simulink model "Cellmodel"  (Simulink 6.6)
settings: Solver=ode4  StartTime=0.0  StopTime=0.0001  FixedStep=0.000000001  RelTol=1e-3
(part 2 of 2)

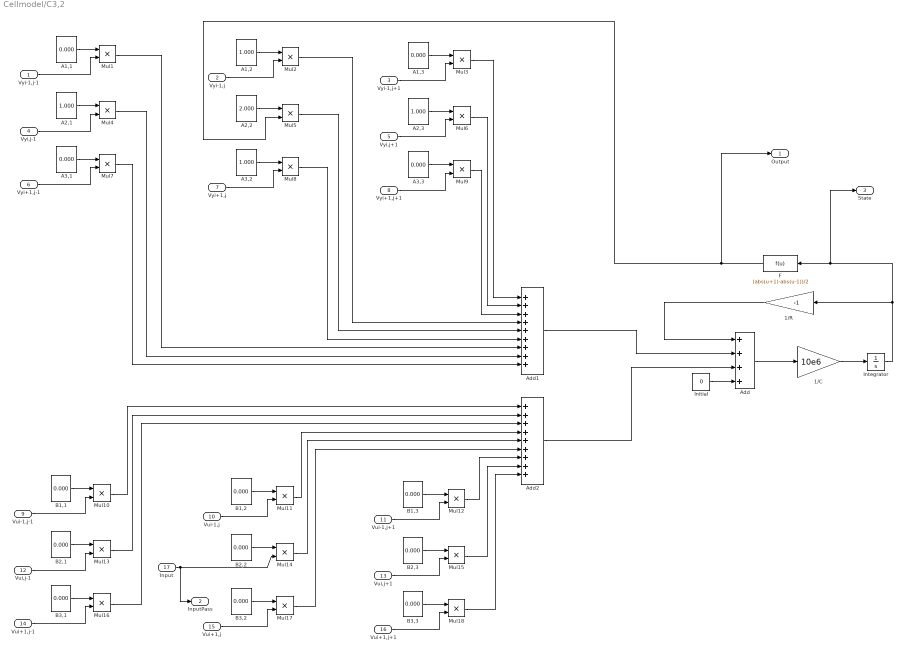
== system Cellmodel/C3,2 ==
  Vyi-1,j-1 : Inport
  Vyi-1,j : Inport  Port=2
  Vyi-1,j+1 : Inport  Port=3
  Vyi,j-1 : Inport  Port=4
  Vyi,j+1 : Inport  Port=5
  Vyi+1,j-1 : Inport  Port=6
  Vyi+1,j : Inport  Port=7
  Vyi+1,j+1 : Inport  Port=8
  Vui-1,j-1 : Inport  Port=9
  Vui-1,j : Inport  Port=10
  Vui-1,j+1 : Inport  Port=11
  Vui,j-1 : Inport  Port=12
  Vui,j+1 : Inport  Port=13
  Vui+1,j-1 : Inport  Port=14
  Vui+1,j : Inport  Port=15
  Vui+1,j+1 : Inport  Port=16
  Input : Inport  Port=17
  1/C : Gain  Gain=10e6
  1/R : Gain  Orientation=left  Gain=-1
  A1,1 : Constant  Value=0.000
  A1,2 : Constant  Value=1.000
  A1,3 : Constant  Value=0.000
  A2,1 : Constant  Value=1.000
  A2,2 : Constant  Value=2.000
  A2,3 : Constant  Value=1.000
  A3,1 : Constant  Value=0.000
  A3,2 : Constant  Value=1.000
  A3,3 : Constant  Value=0.000
  Add : Sum  Inputs=++++  OutScaling=2^-10
  Add1 : Sum  Inputs=+++++++++  OutScaling=2^-10
  Add2 : Sum  Inputs=+++++++++  OutScaling=2^-10
  B1,1 : Constant  Value=0.000
  B1,2 : Constant  Value=0.000
  B1,3 : Constant  Value=0.000
  B2,1 : Constant  Value=0.000
  B2,2 : Constant  Value=0.000
  B2,3 : Constant  Value=0.000
  B3,1 : Constant  Value=0.000
  B3,2 : Constant  Value=0.000
  B3,3 : Constant  Value=0.000
  F : Fcn  Orientation=left  Expr=(abs(u+1)-abs(u-1))/2
  Initial : Constant  Value=0
  Integrator : Integrator  InitialCondition=0.900
  Mul{1..18} (18 alike) : Product  Inputs=**  OutScaling=2^-10
  Output : Outport
  InputPass : Outport  Port=2
  State : Outport  Port=3
  wires:
  Add2/1 -> Add/3
  Input/1 -> InputPass/1, Mul14/2
  Mul18/1 -> Add2/9
  Mul15/1 -> Add2/8
  Mul12/1 -> Add2/7
  Mul17/1 -> Add2/6
  Mul14/1 -> Add2/5
  Mul11/1 -> Add2/4
  Mul16/1 -> Add2/3
  Mul13/1 -> Add2/2
  Mul10/1 -> Add2/1
  Vui+1,j+1/1 -> Mul18/2
  B3,3/1 -> Mul18/1
  Vui+1,j/1 -> Mul17/2
  B3,2/1 -> Mul17/1
  Vui+1,j-1/1 -> Mul16/2
  B3,1/1 -> Mul16/1
  Vui,j+1/1 -> Mul15/2
  B2,3/1 -> Mul15/1
  B2,2/1 -> Mul14/1
  Vui,j-1/1 -> Mul13/2
  B2,1/1 -> Mul13/1
  Vui-1,j+1/1 -> Mul12/2
  B1,3/1 -> Mul12/1
  Vui-1,j/1 -> Mul11/2
  B1,2/1 -> Mul11/1
  Vui-1,j-1/1 -> Mul10/2
  B1,1/1 -> Mul10/1
  Add1/1 -> Add/2
  Mul7/1 -> Add1/9
  Mul4/1 -> Add1/8
  Mul1/1 -> Add1/7
  Mul8/1 -> Add1/6
  Mul5/1 -> Add1/5
  Mul2/1 -> Add1/4
  Mul9/1 -> Add1/3
  Mul6/1 -> Add1/2
  Mul3/1 -> Add1/1
  F/1 -> Mul5/2, Output/1
  Vyi+1,j+1/1 -> Mul9/2
  A3,3/1 -> Mul9/1
  Vyi+1,j/1 -> Mul8/2
  A3,2/1 -> Mul8/1
  Vyi+1,j-1/1 -> Mul7/2
  A3,1/1 -> Mul7/1
  Vyi,j+1/1 -> Mul6/2
  A2,3/1 -> Mul6/1
  A2,2/1 -> Mul5/1
  Vyi,j-1/1 -> Mul4/2
  A2,1/1 -> Mul4/1
  Vyi-1,j+1/1 -> Mul3/2
  A1,3/1 -> Mul3/1
  Vyi-1,j/1 -> Mul2/2
  A1,2/1 -> Mul2/1
  Vyi-1,j-1/1 -> Mul1/2
  A1,1/1 -> Mul1/1
  Integrator/1 -> 1/R/1, F/1, State/1
  1/R/1 -> Add/1
  Initial/1 -> Add/4
  1/C/1 -> Integrator/1
  Add/1 -> 1/C/1

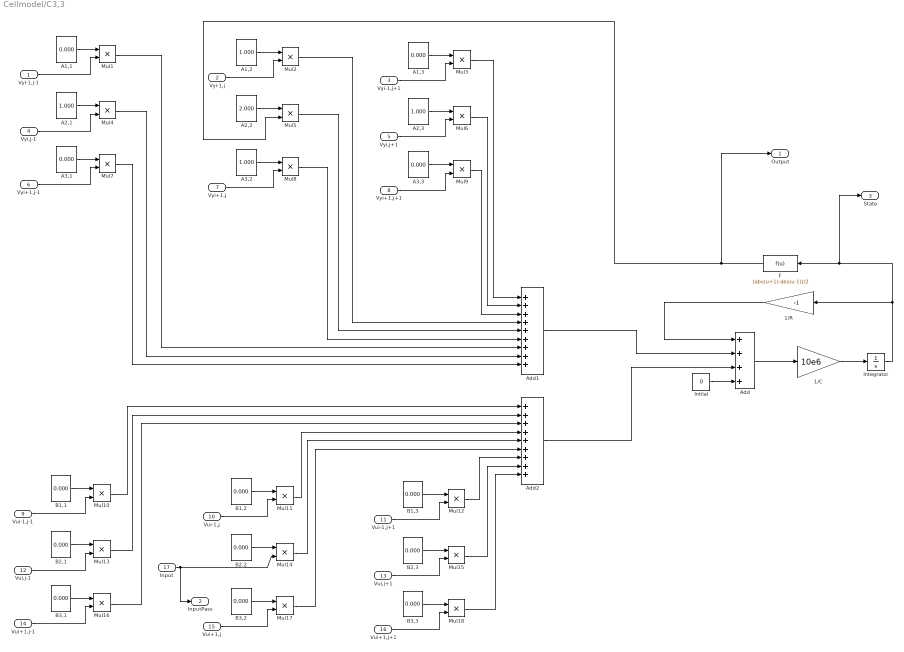
== system Cellmodel/C3,3 ==
  Vyi-1,j-1 : Inport
  Vyi-1,j : Inport  Port=2
  Vyi-1,j+1 : Inport  Port=3
  Vyi,j-1 : Inport  Port=4
  Vyi,j+1 : Inport  Port=5
  Vyi+1,j-1 : Inport  Port=6
  Vyi+1,j : Inport  Port=7
  Vyi+1,j+1 : Inport  Port=8
  Vui-1,j-1 : Inport  Port=9
  Vui-1,j : Inport  Port=10
  Vui-1,j+1 : Inport  Port=11
  Vui,j-1 : Inport  Port=12
  Vui,j+1 : Inport  Port=13
  Vui+1,j-1 : Inport  Port=14
  Vui+1,j : Inport  Port=15
  Vui+1,j+1 : Inport  Port=16
  Input : Inport  Port=17
  1/C : Gain  Gain=10e6
  1/R : Gain  Orientation=left  Gain=-1
  A1,1 : Constant  Value=0.000
  A1,2 : Constant  Value=1.000
  A1,3 : Constant  Value=0.000
  A2,1 : Constant  Value=1.000
  A2,2 : Constant  Value=2.000
  A2,3 : Constant  Value=1.000
  A3,1 : Constant  Value=0.000
  A3,2 : Constant  Value=1.000
  A3,3 : Constant  Value=0.000
  Add : Sum  Inputs=++++  OutScaling=2^-10
  Add1 : Sum  Inputs=+++++++++  OutScaling=2^-10
  Add2 : Sum  Inputs=+++++++++  OutScaling=2^-10
  B1,1 : Constant  Value=0.000
  B1,2 : Constant  Value=0.000
  B1,3 : Constant  Value=0.000
  B2,1 : Constant  Value=0.000
  B2,2 : Constant  Value=0.000
  B2,3 : Constant  Value=0.000
  B3,1 : Constant  Value=0.000
  B3,2 : Constant  Value=0.000
  B3,3 : Constant  Value=0.000
  F : Fcn  Orientation=left  Expr=(abs(u+1)-abs(u-1))/2
  Initial : Constant  Value=0
  Integrator : Integrator  InitialCondition=-1.000
  Mul{1..18} (18 alike) : Product  Inputs=**  OutScaling=2^-10
  Output : Outport
  InputPass : Outport  Port=2
  State : Outport  Port=3
  wires:
  Add/1 -> 1/C/1
  1/C/1 -> Integrator/1
  Initial/1 -> Add/4
  1/R/1 -> Add/1
  Integrator/1 -> 1/R/1, F/1, State/1
  A1,1/1 -> Mul1/1
  Vyi-1,j-1/1 -> Mul1/2
  A1,2/1 -> Mul2/1
  Vyi-1,j/1 -> Mul2/2
  A1,3/1 -> Mul3/1
  Vyi-1,j+1/1 -> Mul3/2
  A2,1/1 -> Mul4/1
  Vyi,j-1/1 -> Mul4/2
  A2,2/1 -> Mul5/1
  A2,3/1 -> Mul6/1
  Vyi,j+1/1 -> Mul6/2
  A3,1/1 -> Mul7/1
  Vyi+1,j-1/1 -> Mul7/2
  A3,2/1 -> Mul8/1
  Vyi+1,j/1 -> Mul8/2
  A3,3/1 -> Mul9/1
  Vyi+1,j+1/1 -> Mul9/2
  F/1 -> Mul5/2, Output/1
  Mul3/1 -> Add1/1
  Mul6/1 -> Add1/2
  Mul9/1 -> Add1/3
  Mul2/1 -> Add1/4
  Mul5/1 -> Add1/5
  Mul8/1 -> Add1/6
  Mul1/1 -> Add1/7
  Mul4/1 -> Add1/8
  Mul7/1 -> Add1/9
  Add1/1 -> Add/2
  B1,1/1 -> Mul10/1
  Vui-1,j-1/1 -> Mul10/2
  B1,2/1 -> Mul11/1
  Vui-1,j/1 -> Mul11/2
  B1,3/1 -> Mul12/1
  Vui-1,j+1/1 -> Mul12/2
  B2,1/1 -> Mul13/1
  Vui,j-1/1 -> Mul13/2
  B2,2/1 -> Mul14/1
  B2,3/1 -> Mul15/1
  Vui,j+1/1 -> Mul15/2
  B3,1/1 -> Mul16/1
  Vui+1,j-1/1 -> Mul16/2
  B3,2/1 -> Mul17/1
  Vui+1,j/1 -> Mul17/2
  B3,3/1 -> Mul18/1
  Vui+1,j+1/1 -> Mul18/2
  Mul10/1 -> Add2/1
  Mul13/1 -> Add2/2
  Mul16/1 -> Add2/3
  Mul11/1 -> Add2/4
  Mul14/1 -> Add2/5
  Mul17/1 -> Add2/6
  Mul12/1 -> Add2/7
  Mul15/1 -> Add2/8
  Mul18/1 -> Add2/9
  Input/1 -> Mul14/2, InputPass/1
  Add2/1 -> Add/3

== system Cellmodel/C3,4 ==
  Vyi-1,j-1 : Inport
  Vyi-1,j : Inport  Port=2
  Vyi-1,j+1 : Inport  Port=3
  Vyi,j-1 : Inport  Port=4
  Vyi,j+1 : Inport  Port=5
  Vyi+1,j-1 : Inport  Port=6
  Vyi+1,j : Inport  Port=7
  Vyi+1,j+1 : Inport  Port=8
  Vui-1,j-1 : Inport  Port=9
  Vui-1,j : Inport  Port=10
  Vui-1,j+1 : Inport  Port=11
  Vui,j-1 : Inport  Port=12
  Vui,j+1 : Inport  Port=13
  Vui+1,j-1 : Inport  Port=14
  Vui+1,j : Inport  Port=15
  Vui+1,j+1 : Inport  Port=16
  Input : Inport  Port=17
  1/C : Gain  Gain=10e6
  1/R : Gain  Orientation=left  Gain=-1
  A1,1 : Constant  Value=0.000
  A1,2 : Constant  Value=1.000
  A1,3 : Constant  Value=0.000
  A2,1 : Constant  Value=1.000
  A2,2 : Constant  Value=2.000
  A2,3 : Constant  Value=1.000
  A3,1 : Constant  Value=0.000
  A3,2 : Constant  Value=1.000
  A3,3 : Constant  Value=0.000
  Add : Sum  Inputs=++++  OutScaling=2^-10
  Add1 : Sum  Inputs=+++++++++  OutScaling=2^-10
  Add2 : Sum  Inputs=+++++++++  OutScaling=2^-10
  B1,1 : Constant  Value=0.000
  B1,2 : Constant  Value=0.000
  B1,3 : Constant  Value=0.000
  B2,1 : Constant  Value=0.000
  B2,2 : Constant  Value=0.000
  B2,3 : Constant  Value=0.000
  B3,1 : Constant  Value=0.000
  B3,2 : Constant  Value=0.000
  B3,3 : Constant  Value=0.000
  F : Fcn  Orientation=left  Expr=(abs(u+1)-abs(u-1))/2
  Initial : Constant  Value=0
  Integrator : Integrator  InitialCondition=-0.800
  Mul{1..18} (18 alike) : Product  Inputs=**  OutScaling=2^-10
  Output : Outport
  InputPass : Outport  Port=2
  State : Outport  Port=3
  wires:
  Add2/1 -> Add/3
  Input/1 -> InputPass/1, Mul14/2
  Mul18/1 -> Add2/9
  Mul15/1 -> Add2/8
  Mul12/1 -> Add2/7
  Mul17/1 -> Add2/6
  Mul14/1 -> Add2/5
  Mul11/1 -> Add2/4
  Mul16/1 -> Add2/3
  Mul13/1 -> Add2/2
  Mul10/1 -> Add2/1
  Vui+1,j+1/1 -> Mul18/2
  B3,3/1 -> Mul18/1
  Vui+1,j/1 -> Mul17/2
  B3,2/1 -> Mul17/1
  Vui+1,j-1/1 -> Mul16/2
  B3,1/1 -> Mul16/1
  Vui,j+1/1 -> Mul15/2
  B2,3/1 -> Mul15/1
  B2,2/1 -> Mul14/1
  Vui,j-1/1 -> Mul13/2
  B2,1/1 -> Mul13/1
  Vui-1,j+1/1 -> Mul12/2
  B1,3/1 -> Mul12/1
  Vui-1,j/1 -> Mul11/2
  B1,2/1 -> Mul11/1
  Vui-1,j-1/1 -> Mul10/2
  B1,1/1 -> Mul10/1
  Add1/1 -> Add/2
  Mul7/1 -> Add1/9
  Mul4/1 -> Add1/8
  Mul1/1 -> Add1/7
  Mul8/1 -> Add1/6
  Mul5/1 -> Add1/5
  Mul2/1 -> Add1/4
  Mul9/1 -> Add1/3
  Mul6/1 -> Add1/2
  Mul3/1 -> Add1/1
  F/1 -> Mul5/2, Output/1
  Vyi+1,j+1/1 -> Mul9/2
  A3,3/1 -> Mul9/1
  Vyi+1,j/1 -> Mul8/2
  A3,2/1 -> Mul8/1
  Vyi+1,j-1/1 -> Mul7/2
  A3,1/1 -> Mul7/1
  Vyi,j+1/1 -> Mul6/2
  A2,3/1 -> Mul6/1
  A2,2/1 -> Mul5/1
  Vyi,j-1/1 -> Mul4/2
  A2,1/1 -> Mul4/1
  Vyi-1,j+1/1 -> Mul3/2
  A1,3/1 -> Mul3/1
  Vyi-1,j/1 -> Mul2/2
  A1,2/1 -> Mul2/1
  Vyi-1,j-1/1 -> Mul1/2
  A1,1/1 -> Mul1/1
  Integrator/1 -> 1/R/1, F/1, State/1
  1/R/1 -> Add/1
  Initial/1 -> Add/4
  1/C/1 -> Integrator/1
  Add/1 -> 1/C/1

== system Cellmodel/C4,1 ==
  Vyi-1,j-1 : Inport
  Vyi-1,j : Inport  Port=2
  Vyi-1,j+1 : Inport  Port=3
  Vyi,j-1 : Inport  Port=4
  Vyi,j+1 : Inport  Port=5
  Vyi+1,j-1 : Inport  Port=6
  Vyi+1,j : Inport  Port=7
  Vyi+1,j+1 : Inport  Port=8
  Vui-1,j-1 : Inport  Port=9
  Vui-1,j : Inport  Port=10
  Vui-1,j+1 : Inport  Port=11
  Vui,j-1 : Inport  Port=12
  Vui,j+1 : Inport  Port=13
  Vui+1,j-1 : Inport  Port=14
  Vui+1,j : Inport  Port=15
  Vui+1,j+1 : Inport  Port=16
  Input : Inport  Port=17
  1/C : Gain  Gain=10e6
  1/R : Gain  Orientation=left  Gain=-1
  A1,1 : Constant  Value=0.000
  A1,2 : Constant  Value=1.000
  A1,3 : Constant  Value=0.000
  A2,1 : Constant  Value=1.000
  A2,2 : Constant  Value=2.000
  A2,3 : Constant  Value=1.000
  A3,1 : Constant  Value=0.000
  A3,2 : Constant  Value=1.000
  A3,3 : Constant  Value=0.000
  Add : Sum  Inputs=++++  OutScaling=2^-10
  Add1 : Sum  Inputs=+++++++++  OutScaling=2^-10
  Add2 : Sum  Inputs=+++++++++  OutScaling=2^-10
  B1,1 : Constant  Value=0.000
  B1,2 : Constant  Value=0.000
  B1,3 : Constant  Value=0.000
  B2,1 : Constant  Value=0.000
  B2,2 : Constant  Value=0.000
  B2,3 : Constant  Value=0.000
  B3,1 : Constant  Value=0.000
  B3,2 : Constant  Value=0.000
  B3,3 : Constant  Value=0.000
  F : Fcn  Orientation=left  Expr=(abs(u+1)-abs(u-1))/2
  Initial : Constant  Value=0
  Integrator : Integrator  InitialCondition=-0.900
  Mul{1..18} (18 alike) : Product  Inputs=**  OutScaling=2^-10
  Output : Outport
  InputPass : Outport  Port=2
  State : Outport  Port=3
  wires:
  Add2/1 -> Add/3
  Input/1 -> InputPass/1, Mul14/2
  Mul18/1 -> Add2/9
  Mul15/1 -> Add2/8
  Mul12/1 -> Add2/7
  Mul17/1 -> Add2/6
  Mul14/1 -> Add2/5
  Mul11/1 -> Add2/4
  Mul16/1 -> Add2/3
  Mul13/1 -> Add2/2
  Mul10/1 -> Add2/1
  Vui+1,j+1/1 -> Mul18/2
  B3,3/1 -> Mul18/1
  Vui+1,j/1 -> Mul17/2
  B3,2/1 -> Mul17/1
  Vui+1,j-1/1 -> Mul16/2
  B3,1/1 -> Mul16/1
  Vui,j+1/1 -> Mul15/2
  B2,3/1 -> Mul15/1
  B2,2/1 -> Mul14/1
  Vui,j-1/1 -> Mul13/2
  B2,1/1 -> Mul13/1
  Vui-1,j+1/1 -> Mul12/2
  B1,3/1 -> Mul12/1
  Vui-1,j/1 -> Mul11/2
  B1,2/1 -> Mul11/1
  Vui-1,j-1/1 -> Mul10/2
  B1,1/1 -> Mul10/1
  Add1/1 -> Add/2
  Mul7/1 -> Add1/9
  Mul4/1 -> Add1/8
  Mul1/1 -> Add1/7
  Mul8/1 -> Add1/6
  Mul5/1 -> Add1/5
  Mul2/1 -> Add1/4
  Mul9/1 -> Add1/3
  Mul6/1 -> Add1/2
  Mul3/1 -> Add1/1
  F/1 -> Mul5/2, Output/1
  Vyi+1,j+1/1 -> Mul9/2
  A3,3/1 -> Mul9/1
  Vyi+1,j/1 -> Mul8/2
  A3,2/1 -> Mul8/1
  Vyi+1,j-1/1 -> Mul7/2
  A3,1/1 -> Mul7/1
  Vyi,j+1/1 -> Mul6/2
  A2,3/1 -> Mul6/1
  A2,2/1 -> Mul5/1
  Vyi,j-1/1 -> Mul4/2
  A2,1/1 -> Mul4/1
  Vyi-1,j+1/1 -> Mul3/2
  A1,3/1 -> Mul3/1
  Vyi-1,j/1 -> Mul2/2
  A1,2/1 -> Mul2/1
  Vyi-1,j-1/1 -> Mul1/2
  A1,1/1 -> Mul1/1
  Integrator/1 -> 1/R/1, F/1, State/1
  1/R/1 -> Add/1
  Initial/1 -> Add/4
  1/C/1 -> Integrator/1
  Add/1 -> 1/C/1

== system Cellmodel/C4,2 ==
  Vyi-1,j-1 : Inport
  Vyi-1,j : Inport  Port=2
  Vyi-1,j+1 : Inport  Port=3
  Vyi,j-1 : Inport  Port=4
  Vyi,j+1 : Inport  Port=5
  Vyi+1,j-1 : Inport  Port=6
  Vyi+1,j : Inport  Port=7
  Vyi+1,j+1 : Inport  Port=8
  Vui-1,j-1 : Inport  Port=9
  Vui-1,j : Inport  Port=10
  Vui-1,j+1 : Inport  Port=11
  Vui,j-1 : Inport  Port=12
  Vui,j+1 : Inport  Port=13
  Vui+1,j-1 : Inport  Port=14
  Vui+1,j : Inport  Port=15
  Vui+1,j+1 : Inport  Port=16
  Input : Inport  Port=17
  1/C : Gain  Gain=10e6
  1/R : Gain  Orientation=left  Gain=-1
  A1,1 : Constant  Value=0.000
  A1,2 : Constant  Value=1.000
  A1,3 : Constant  Value=0.000
  A2,1 : Constant  Value=1.000
  A2,2 : Constant  Value=2.000
  A2,3 : Constant  Value=1.000
  A3,1 : Constant  Value=0.000
  A3,2 : Constant  Value=1.000
  A3,3 : Constant  Value=0.000
  Add : Sum  Inputs=++++  OutScaling=2^-10
  Add1 : Sum  Inputs=+++++++++  OutScaling=2^-10
  Add2 : Sum  Inputs=+++++++++  OutScaling=2^-10
  B1,1 : Constant  Value=0.000
  B1,2 : Constant  Value=0.000
  B1,3 : Constant  Value=0.000
  B2,1 : Constant  Value=0.000
  B2,2 : Constant  Value=0.000
  B2,3 : Constant  Value=0.000
  B3,1 : Constant  Value=0.000
  B3,2 : Constant  Value=0.000
  B3,3 : Constant  Value=0.000
  F : Fcn  Orientation=left  Expr=(abs(u+1)-abs(u-1))/2
  Initial : Constant  Value=0
  Integrator : Integrator  InitialCondition=-1.000
  Mul{1..18} (18 alike) : Product  Inputs=**  OutScaling=2^-10
  Output : Outport
  InputPass : Outport  Port=2
  State : Outport  Port=3
  wires:
  Add/1 -> 1/C/1
  1/C/1 -> Integrator/1
  Initial/1 -> Add/4
  1/R/1 -> Add/1
  Integrator/1 -> 1/R/1, F/1, State/1
  A1,1/1 -> Mul1/1
  Vyi-1,j-1/1 -> Mul1/2
  A1,2/1 -> Mul2/1
  Vyi-1,j/1 -> Mul2/2
  A1,3/1 -> Mul3/1
  Vyi-1,j+1/1 -> Mul3/2
  A2,1/1 -> Mul4/1
  Vyi,j-1/1 -> Mul4/2
  A2,2/1 -> Mul5/1
  A2,3/1 -> Mul6/1
  Vyi,j+1/1 -> Mul6/2
  A3,1/1 -> Mul7/1
  Vyi+1,j-1/1 -> Mul7/2
  A3,2/1 -> Mul8/1
  Vyi+1,j/1 -> Mul8/2
  A3,3/1 -> Mul9/1
  Vyi+1,j+1/1 -> Mul9/2
  F/1 -> Mul5/2, Output/1
  Mul3/1 -> Add1/1
  Mul6/1 -> Add1/2
  Mul9/1 -> Add1/3
  Mul2/1 -> Add1/4
  Mul5/1 -> Add1/5
  Mul8/1 -> Add1/6
  Mul1/1 -> Add1/7
  Mul4/1 -> Add1/8
  Mul7/1 -> Add1/9
  Add1/1 -> Add/2
  B1,1/1 -> Mul10/1
  Vui-1,j-1/1 -> Mul10/2
  B1,2/1 -> Mul11/1
  Vui-1,j/1 -> Mul11/2
  B1,3/1 -> Mul12/1
  Vui-1,j+1/1 -> Mul12/2
  B2,1/1 -> Mul13/1
  Vui,j-1/1 -> Mul13/2
  B2,2/1 -> Mul14/1
  B2,3/1 -> Mul15/1
  Vui,j+1/1 -> Mul15/2
  B3,1/1 -> Mul16/1
  Vui+1,j-1/1 -> Mul16/2
  B3,2/1 -> Mul17/1
  Vui+1,j/1 -> Mul17/2
  B3,3/1 -> Mul18/1
  Vui+1,j+1/1 -> Mul18/2
  Mul10/1 -> Add2/1
  Mul13/1 -> Add2/2
  Mul16/1 -> Add2/3
  Mul11/1 -> Add2/4
  Mul14/1 -> Add2/5
  Mul17/1 -> Add2/6
  Mul12/1 -> Add2/7
  Mul15/1 -> Add2/8
  Mul18/1 -> Add2/9
  Input/1 -> Mul14/2, InputPass/1
  Add2/1 -> Add/3

== system Cellmodel/C4,3 ==
  Vyi-1,j-1 : Inport
  Vyi-1,j : Inport  Port=2
  Vyi-1,j+1 : Inport  Port=3
  Vyi,j-1 : Inport  Port=4
  Vyi,j+1 : Inport  Port=5
  Vyi+1,j-1 : Inport  Port=6
  Vyi+1,j : Inport  Port=7
  Vyi+1,j+1 : Inport  Port=8
  Vui-1,j-1 : Inport  Port=9
  Vui-1,j : Inport  Port=10
  Vui-1,j+1 : Inport  Port=11
  Vui,j-1 : Inport  Port=12
  Vui,j+1 : Inport  Port=13
  Vui+1,j-1 : Inport  Port=14
  Vui+1,j : Inport  Port=15
  Vui+1,j+1 : Inport  Port=16
  Input : Inport  Port=17
  1/C : Gain  Gain=10e6
  1/R : Gain  Orientation=left  Gain=-1
  A1,1 : Constant  Value=0.000
  A1,2 : Constant  Value=1.000
  A1,3 : Constant  Value=0.000
  A2,1 : Constant  Value=1.000
  A2,2 : Constant  Value=2.000
  A2,3 : Constant  Value=1.000
  A3,1 : Constant  Value=0.000
  A3,2 : Constant  Value=1.000
  A3,3 : Constant  Value=0.000
  Add : Sum  Inputs=++++  OutScaling=2^-10
  Add1 : Sum  Inputs=+++++++++  OutScaling=2^-10
  Add2 : Sum  Inputs=+++++++++  OutScaling=2^-10
  B1,1 : Constant  Value=0.000
  B1,2 : Constant  Value=0.000
  B1,3 : Constant  Value=0.000
  B2,1 : Constant  Value=0.000
  B2,2 : Constant  Value=0.000
  B2,3 : Constant  Value=0.000
  B3,1 : Constant  Value=0.000
  B3,2 : Constant  Value=0.000
  B3,3 : Constant  Value=0.000
  F : Fcn  Orientation=left  Expr=(abs(u+1)-abs(u-1))/2
  Initial : Constant  Value=0
  Integrator : Integrator  InitialCondition=-0.700
  Mul{1..18} (18 alike) : Product  Inputs=**  OutScaling=2^-10
  Output : Outport
  InputPass : Outport  Port=2
  State : Outport  Port=3
  wires:
  Add2/1 -> Add/3
  Input/1 -> InputPass/1, Mul14/2
  Mul18/1 -> Add2/9
  Mul15/1 -> Add2/8
  Mul12/1 -> Add2/7
  Mul17/1 -> Add2/6
  Mul14/1 -> Add2/5
  Mul11/1 -> Add2/4
  Mul16/1 -> Add2/3
  Mul13/1 -> Add2/2
  Mul10/1 -> Add2/1
  Vui+1,j+1/1 -> Mul18/2
  B3,3/1 -> Mul18/1
  Vui+1,j/1 -> Mul17/2
  B3,2/1 -> Mul17/1
  Vui+1,j-1/1 -> Mul16/2
  B3,1/1 -> Mul16/1
  Vui,j+1/1 -> Mul15/2
  B2,3/1 -> Mul15/1
  B2,2/1 -> Mul14/1
  Vui,j-1/1 -> Mul13/2
  B2,1/1 -> Mul13/1
  Vui-1,j+1/1 -> Mul12/2
  B1,3/1 -> Mul12/1
  Vui-1,j/1 -> Mul11/2
  B1,2/1 -> Mul11/1
  Vui-1,j-1/1 -> Mul10/2
  B1,1/1 -> Mul10/1
  Add1/1 -> Add/2
  Mul7/1 -> Add1/9
  Mul4/1 -> Add1/8
  Mul1/1 -> Add1/7
  Mul8/1 -> Add1/6
  Mul5/1 -> Add1/5
  Mul2/1 -> Add1/4
  Mul9/1 -> Add1/3
  Mul6/1 -> Add1/2
  Mul3/1 -> Add1/1
  F/1 -> Mul5/2, Output/1
  Vyi+1,j+1/1 -> Mul9/2
  A3,3/1 -> Mul9/1
  Vyi+1,j/1 -> Mul8/2
  A3,2/1 -> Mul8/1
  Vyi+1,j-1/1 -> Mul7/2
  A3,1/1 -> Mul7/1
  Vyi,j+1/1 -> Mul6/2
  A2,3/1 -> Mul6/1
  A2,2/1 -> Mul5/1
  Vyi,j-1/1 -> Mul4/2
  A2,1/1 -> Mul4/1
  Vyi-1,j+1/1 -> Mul3/2
  A1,3/1 -> Mul3/1
  Vyi-1,j/1 -> Mul2/2
  A1,2/1 -> Mul2/1
  Vyi-1,j-1/1 -> Mul1/2
  A1,1/1 -> Mul1/1
  Integrator/1 -> 1/R/1, F/1, State/1
  1/R/1 -> Add/1
  Initial/1 -> Add/4
  1/C/1 -> Integrator/1
  Add/1 -> 1/C/1

== system Cellmodel/C4,4 ==
  Vyi-1,j-1 : Inport
  Vyi-1,j : Inport  Port=2
  Vyi-1,j+1 : Inport  Port=3
  Vyi,j-1 : Inport  Port=4
  Vyi,j+1 : Inport  Port=5
  Vyi+1,j-1 : Inport  Port=6
  Vyi+1,j : Inport  Port=7
  Vyi+1,j+1 : Inport  Port=8
  Vui-1,j-1 : Inport  Port=9
  Vui-1,j : Inport  Port=10
  Vui-1,j+1 : Inport  Port=11
  Vui,j-1 : Inport  Port=12
  Vui,j+1 : Inport  Port=13
  Vui+1,j-1 : Inport  Port=14
  Vui+1,j : Inport  Port=15
  Vui+1,j+1 : Inport  Port=16
  Input : Inport  Port=17
  1/C : Gain  Gain=10e6
  1/R : Gain  Orientation=left  Gain=-1
  A1,1 : Constant  Value=0.000
  A1,2 : Constant  Value=1.000
  A1,3 : Constant  Value=0.000
  A2,1 : Constant  Value=1.000
  A2,2 : Constant  Value=2.000
  A2,3 : Constant  Value=1.000
  A3,1 : Constant  Value=0.000
  A3,2 : Constant  Value=1.000
  A3,3 : Constant  Value=0.000
  Add : Sum  Inputs=++++  OutScaling=2^-10
  Add1 : Sum  Inputs=+++++++++  OutScaling=2^-10
  Add2 : Sum  Inputs=+++++++++  OutScaling=2^-10
  B1,1 : Constant  Value=0.000
  B1,2 : Constant  Value=0.000
  B1,3 : Constant  Value=0.000
  B2,1 : Constant  Value=0.000
  B2,2 : Constant  Value=0.000
  B2,3 : Constant  Value=0.000
  B3,1 : Constant  Value=0.000
  B3,2 : Constant  Value=0.000
  B3,3 : Constant  Value=0.000
  F : Fcn  Orientation=left  Expr=(abs(u+1)-abs(u-1))/2
  Initial : Constant  Value=0
  Integrator : Integrator  InitialCondition=-0.800
  Mul{1..18} (18 alike) : Product  Inputs=**  OutScaling=2^-10
  Output : Outport
  InputPass : Outport  Port=2
  State : Outport  Port=3
  wires:
  Add/1 -> 1/C/1
  1/C/1 -> Integrator/1
  Initial/1 -> Add/4
  1/R/1 -> Add/1
  Integrator/1 -> 1/R/1, F/1, State/1
  A1,1/1 -> Mul1/1
  Vyi-1,j-1/1 -> Mul1/2
  A1,2/1 -> Mul2/1
  Vyi-1,j/1 -> Mul2/2
  A1,3/1 -> Mul3/1
  Vyi-1,j+1/1 -> Mul3/2
  A2,1/1 -> Mul4/1
  Vyi,j-1/1 -> Mul4/2
  A2,2/1 -> Mul5/1
  A2,3/1 -> Mul6/1
  Vyi,j+1/1 -> Mul6/2
  A3,1/1 -> Mul7/1
  Vyi+1,j-1/1 -> Mul7/2
  A3,2/1 -> Mul8/1
  Vyi+1,j/1 -> Mul8/2
  A3,3/1 -> Mul9/1
  Vyi+1,j+1/1 -> Mul9/2
  F/1 -> Mul5/2, Output/1
  Mul3/1 -> Add1/1
  Mul6/1 -> Add1/2
  Mul9/1 -> Add1/3
  Mul2/1 -> Add1/4
  Mul5/1 -> Add1/5
  Mul8/1 -> Add1/6
  Mul1/1 -> Add1/7
  Mul4/1 -> Add1/8
  Mul7/1 -> Add1/9
  Add1/1 -> Add/2
  B1,1/1 -> Mul10/1
  Vui-1,j-1/1 -> Mul10/2
  B1,2/1 -> Mul11/1
  Vui-1,j/1 -> Mul11/2
  B1,3/1 -> Mul12/1
  Vui-1,j+1/1 -> Mul12/2
  B2,1/1 -> Mul13/1
  Vui,j-1/1 -> Mul13/2
  B2,2/1 -> Mul14/1
  B2,3/1 -> Mul15/1
  Vui,j+1/1 -> Mul15/2
  B3,1/1 -> Mul16/1
  Vui+1,j-1/1 -> Mul16/2
  B3,2/1 -> Mul17/1
  Vui+1,j/1 -> Mul17/2
  B3,3/1 -> Mul18/1
  Vui+1,j+1/1 -> Mul18/2
  Mul10/1 -> Add2/1
  Mul13/1 -> Add2/2
  Mul16/1 -> Add2/3
  Mul11/1 -> Add2/4
  Mul14/1 -> Add2/5
  Mul17/1 -> Add2/6
  Mul12/1 -> Add2/7
  Mul15/1 -> Add2/8
  Mul18/1 -> Add2/9
  Input/1 -> Mul14/2, InputPass/1
  Add2/1 -> Add/3
